simulink model "LKATestBenchExample_sthBrokeGoddamned"  (R2020b)
settings: Solver=FixedStepAuto  StartTime=0.0  StopTime=simStopTime  RelTol=1e-3
PostLoadFcn:
  | helperLKASetUp
values from neighbouring files (symbols this model uses):
  lr = 1.2    [Model_Init.m]    (also in Model_Init_Varying.m; helperLKASetUp.m = 1.6; helperLKASetUpVarying.m = 1.6; modelInit.m)
  m = 1575    [Model_Init.m]    (also in Model_Init_Varying.m; helperLKASetUp.m; helperLKASetUpVarying.m; modelInit.m)
  v = 20    [LVI_PDNN_for_QP_init.m]    (also in Model_Init_Varying.m = 15; automatedBayes.m = i; runSimOnce.m = 36)
  v0_ego = Vx    [Model_Init.m]    (also in Model_Init_Varying.m = 15)
  yaw0_ego = 0    [BayesOpt.m]    (also in helperLKASetUpVarying.m = -90)
undefined symbols (not defined in the file or in its folder): Curvature, CurvatureDerivative, driverPath, driving, HeadingAngle, LateralOffset, Left, Right, Strength
libraries: simulink x2, drivingscenarioandsensors x2, pid_lib x1, autolibshared x1
CloseFcn:
  | helperLKACleanUp
settings Model: Creator=The MathWorks, Inc.  LastModifiedBy=Stage
settings DataIOCC: ReturnWorkspaceOutputs=off
settings DebuggingCC: ParameterPrecisionLossMsg=none  ArithmeticOperatorsInVariantConditions=warning
settings HardwareCC: ProdLongLongMode=on
settings SFSimCC: SimUseLocalCustomCode=off
settings RTWCC: RTWUseLocalCustomCode=off

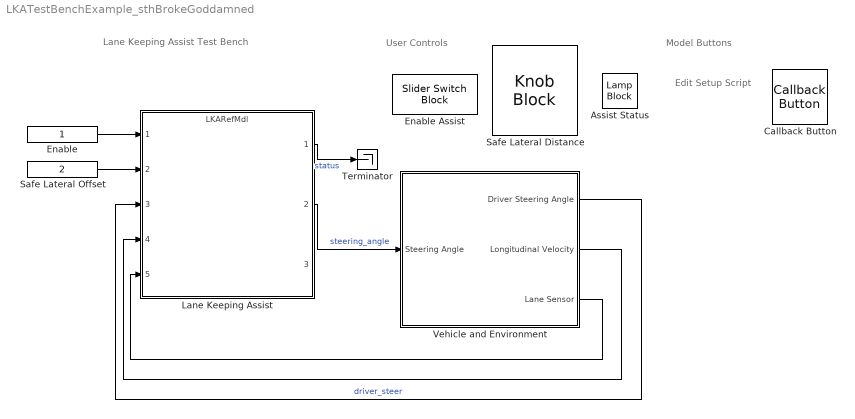
== system LKATestBenchExample_sthBrokeGoddamned ==
  note: User Controls
  note: Edit Setup Script
  note: Lane Keeping Assist Test Bench
  note: Model Buttons
  Assist Status : LampBlock  LabelPosition=Hide
  Callback Button : CallbackButton  ButtonText=?
      settings: ClickFcn=|
      | exampleID = 'LaneKeepingAssistWithLaneDetectionExample';
      | exampleName = 'lane-keeping-assist-with-lane-detection.html';
      | if license('test','automated_driving_toolbox') && ~isempty(ver('driving'))
      |     helpview('driving',exampleID);
      | elseif license('test','MPC_Toolbox') && ~isempty(ver('mpc'))
      |     helpview('mpc',exampleID);
      | else
      |     web(fullfile('https://www.mathworks.com/help','driving','examples',exampleName));
      | end
      | clear exampleName exampleID;
  Enable : Constant  OutDataTypeStr=Inherit: Inherit via back propagation
  Enable Assist : SliderSwitchBlock  LabelPosition=Hide
      settings: Values={{'Off', 'On'}, [0 1]}
  Lane Keeping Assist : ModelReference  ModelNameDialog=LKARefMdl.slx  SimulationMode=Normal  CodeInterface=Top model  ModelReferenceVersion=1.373
  Safe Lateral Distance : KnobBlock  LabelPosition=Hide  ScaleMax=2  TickInterval=0.5
  Safe Lateral Offset : Constant  Value=2  OutDataTypeStr=Inherit: Inherit via back propagation
  Terminator : Terminator
  Vehicle and Environment : Subsystem
  wires:
  Lane Keeping Assist/1 -> Terminator/1  "status"
  Lane Keeping Assist/2 -> Vehicle and Environment/1(Steering Angle)  "steering_angle"
  Enable/1 -> Lane Keeping Assist/1
  Vehicle and Environment/3(Lane Sensor) -> Lane Keeping Assist/5
  Safe Lateral Offset/1 -> Lane Keeping Assist/2
  Vehicle and Environment/1(Driver Steering Angle) -> Lane Keeping Assist/3  "driver_steer"
  Vehicle and Environment/2(Longitudinal Velocity) -> Lane Keeping Assist/4

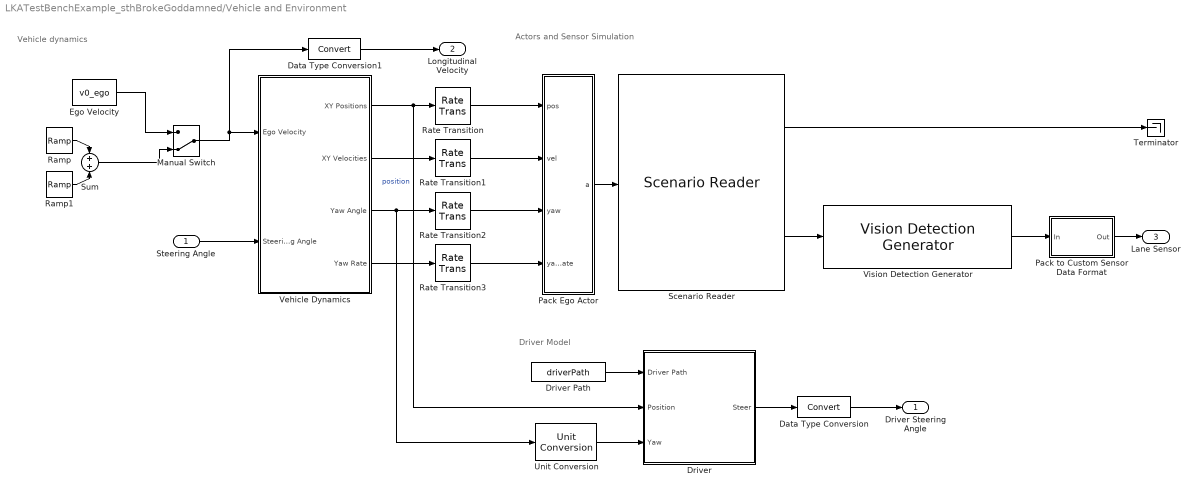
== system LKATestBenchExample_sthBrokeGoddamned/Vehicle and Environment ==
  note: Vehicle dynamics
  note: Actors and Sensor Simulation
  note: Driver Model
  Steering Angle : Inport  Unit=rad
  Data Type Conversion : DataTypeConversion
  Data Type Conversion1 : DataTypeConversion
  Driver : Subsystem
  Driver Path : Constant  Value=driverPath
  Ego Velocity : Constant  Value=v0_ego
  Manual Switch : ManualSwitch  CurrentSetting=0
  Pack Ego Actor : MATLAB Function  TreatAsAtomicUnit=on
  Pack to Custom Sensor Data Format : Subsystem
  Ramp : simulink/Sources/Ramp  slope=-5  start=v/5  InitialOutput=0
  Ramp1 : simulink/Sources/Ramp  slope=5  start=0  InitialOutput=0
  Rate Transition{,1..3} (4 alike) : RateTransition  OutPortSampleTime=Ts
  Scenario Reader : drivingscenarioandsensors/Scenario Reader  ScenarioSource=From workspace  ScenarioFileName=MyDynamicScenario.mat  ScenarioVariableName=scenario1  OutputCoordinateSystem=Vehicle coordinates  EgoVehicleSource=Input port  EgoVehicleActorID=1  OrientVehiclesOnRoad=off  OutputEgoVehiclePose=off  SampleTime=0.1  LaneBoundaryOutput=Ego vehicle lane boundaries  LaneBoundaryDistance=0:0.5:60  LaneBoundaryLocation=Inner edge of lane markings  BusNameSource=Auto  BusName=BusActors  BusName2Source=Auto  BusName2=BusLaneBoundaries  BusName3Source=Auto  BusName3=BusEgoActor  ShowCoordinateLabels=on  SimulateUsing=Interpreted execution
  Sum : Sum  Inputs=+|+
  Terminator : Terminator
  Unit Conversion : UnitConversion
  Vehicle Dynamics : Subsystem  VariantControl=VariantVDBS
  Vision Detection Generator : drivingscenarioandsensors/Vision Detection Generator  SensorIndex=1  DetectorOutput=Lanes only  UpdateInterval=0.1  LaneUpdateInterval=0.1  SensorLocation=[ 1.9, 0 ]  Height=1.1  Yaw=0  Pitch=1  Roll=0  BusNameSource=Auto  BusName=BusObjectDetections  BusName2Source=Property  BusName2=BusVision  MaxNumDetectionsSource=Property  MaxNumDetections=50  MaxNumLanesSource=Property  MaxNumLanes=2  DetectionCoordinates=Ego Cartesian  SimulateUsing=Interpreted execution  MaxRange=150  BoundingBoxAccuracy=5  ProcessNoiseIntensity=5  MaxSpeed=50  MaxAllowedOcclusion=0.5  MinObjectImageSize=[ 15, 15 ]  DetectionProbability=0.9  FalsePositivesPerImage=0.1  MinLaneImageSize=[ 20, 3 ]  LaneBoundaryAccuracy=3  HasNoise=on  InitialSeedSource=Repeatable  InitialSeed=0  UsedSeed=driving.internal.SimulinkUtilities.seedManager(gcb)  ActorProfilesSource=Parameters  ActorProfilesParameters=driving.internal.ActorProfilesParameters  ActorProfilesExpression=struct( 'ClassID', 0, 'Length', 4.7, 'Width', 1.8, 'Height', 1.4, 'OriginOffset', [ -1.35, 0, 0 ] )  Intrinsics=driving.internal.cameraIntrinsics('FocalLength',[ 100, 100 ])
  Driver Steering Angle : Outport  VectorParamsAs1DForOutWhenUnconnected=off
  Longitudinal Velocity : Outport  Port=2  OutDataTypeStr=single  Unit=m/s  VectorParamsAs1DForOutWhenUnconnected=off
  Lane Sensor : Outport  Port=3  VectorParamsAs1DForOutWhenUnconnected=off
  wires:
  Scenario Reader/1 -> Terminator/1
  Pack Ego Actor/1(a) -> Scenario Reader/1
  Vehicle Dynamics/2(XY Velocities) -> Rate Transition1/1
  Vehicle Dynamics/3(Yaw Angle) -> Unit Conversion/1, Rate Transition2/1
  Rate Transition/1 -> Pack Ego Actor/1(pos)
  Vehicle Dynamics/4(Yaw Rate) -> Rate Transition3/1
  Rate Transition2/1 -> Pack Ego Actor/3(yaw)
  Rate Transition1/1 -> Pack Ego Actor/2(vel)
  Rate Transition3/1 -> Pack Ego Actor/4(yawRate)
  Scenario Reader/2 -> Vision Detection Generator/1
  Vehicle Dynamics/1(XY Positions) -> Driver/2(Position), Rate Transition/1  "position"
  Driver/1(Steer) -> Data Type Conversion/1
  Steering Angle/1 -> Vehicle Dynamics/2(Steering Angle)
  Unit Conversion/1 -> Driver/3(Yaw)
  Vision Detection Generator/1 -> Pack to Custom Sensor Data Format/1(In)
  Data Type Conversion/1 -> Driver Steering Angle/1
  Pack to Custom Sensor Data Format/1(Out) -> Lane Sensor/1
  Data Type Conversion1/1 -> Longitudinal Velocity/1
  Driver Path/1 -> Driver/1(Driver Path)
  Ramp1/1 -> Sum/2
  Ramp/1 -> Sum/1
  Ego Velocity/1 -> Manual Switch/1
  Manual Switch/1 -> Data Type Conversion1/1, Vehicle Dynamics/1(Ego Velocity)
  Sum/1 -> Manual Switch/2

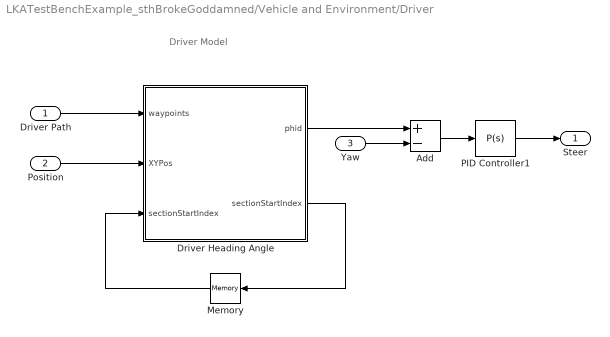
== system LKATestBenchExample_sthBrokeGoddamned/Vehicle and Environment/Driver ==
  note: Driver Model
  Driver Path : Inport  Unit=m
  Position : Inport  Port=2  Unit=m
  Yaw : Inport  Port=3  Unit=rad
  Add : Sum  Inputs=+-
  Driver Heading Angle : MATLAB Function  TreatAsAtomicUnit=on
  Memory : Memory
  PID Controller1 : pid_lib/PID Controller  Controller=P  Form=Parallel  TimeDomain=Continuous-time  UseExternalTs=off  SampleTime=-1  IntegratorMethod=Forward Euler  FilterMethod=Forward Euler  ControllerParametersSource=internal  P=1  I=0.002  D=0.00001  UseFilter=on  N=100  TunerSelectOption=Transfer Function Based (PID Tuner App)  InitialConditionSource=internal  InitialConditionForIntegrator=0  InitialConditionForFilter=0  DifferentiatorICPrevScaledInput=0  ExternalReset=none  TrackingMode=off  Kt=1  LimitOutput=off  SatLimitsSource=internal  UpperSaturationLimit=inf  LowerSaturationLimit=-inf  LinearizeAsGain=on  AntiWindupMode=none  Kb=1  POutMin=[]  POutMax=[]  IOutMin=[]  IOutMax=[]  DOutMin=[]  DOutMax=[]  NOutMin=[]  NOutMax=[]  SumOutMin=[]  SumOutMax=[]  SaturationOutMin=[]  SaturationOutMax=[]  PParamMin=[]  PParamMax=[]  IParamMin=[]  IParamMax=[]  DParamMin=[]  DParamMax=[]  NParamMin=[]  NParamMax=[]  KbParamMin=[]  KbParamMax=[]  KtParamMin=[]  KtParamMax=[]  KbOutMin=[]  KbOutMax=[]  KtOutMin=[]  KtOutMax=[]  IntegratorOutMin=[]  IntegratorOutMax=[]  FilterOutMin=[]  FilterOutMax=[]  SumI1OutMin=[]  SumI1OutMax=[]  SumI2OutMin=[]  SumI2OutMax=[]  SumI3OutMin=[]  SumI3OutMax=[]  SumI4OutMin=[]  SumI4OutMax=[]  SumDOutMin=[]  SumDOutMax=[]  DifferentiatorOutMin=[]  DifferentiatorOutMax=[]  FilterDiffOutCoefMin=[]  FilterDiffOutCoefMax=[]  ReciprocalOutMin=[]  ReciprocalOutMax=[]  SumDenOutMin=[]  SumDenOutMax=[]  SumNumOutMin=[]  SumNumOutMax=[]  DivideOutMin=[]  DivideOutMax=[]  UdiffTsProdOutMin=[]  UdiffTsProdOutMax=[]  NTsProdOutMin=[]  NTsProdOutMax=[]  UintegralTsProdOutMin=[]  UintegralTsProdOutMax=[]  UngainTsProdOutMin=[]  UngainTsProdOutMax=[]  IntegratorContinuousStateAttributes=''  IntegratorStateMustResolveToSignalObject=off  IntegratorRTWStateStorageClass=Auto  FilterContinuousStateAttributes=''  FilterStateMustResolveToSignalObject=off  FilterRTWStateStorageClass=Auto  ParallelPVariant=InternalParameters  IdealPVariant=Disabled  IVariant=Disabled  DVariant=Disabled  IntegratorVariant=Disabled  SatVariant=Disabled  AWVariant=Disabled  PCopyVariant=Disabled  TRVariant=Disabled  FdbkBlocksVariant=Forward  IdealPFdbkVariant=Disabled  SatFdbkVariant=Disabled  DerivativeFilterVariant=Disabled  NVariant=Disabled  NCopyVariant=Disabled_SignalSpec  FilterICVariant=Disabled  IntegratorICVariant=Disabled  ExternalResetVariant=Disabled  TRSumVariant=Passthrough  SumFdbkVariant=Disabled  SumVariant=Passthrough_P  TsampFilterVariant=InternalTs  TsampNgainVariant=Passthrough  TsampIntegralVariant=Disabled_SignalSpec  ExternalSaturationOutDataTypeStr=Inherit: Same as second input
  Steer : Outport  Unit=rad  VectorParamsAs1DForOutWhenUnconnected=off
  wires:
  Yaw/1 -> Add/2
  Position/1 -> Driver Heading Angle/2(XYPos)
  Driver Path/1 -> Driver Heading Angle/1(waypoints)
  Driver Heading Angle/1(phid) -> Add/1
  PID Controller1/1 -> Steer/1
  Driver Heading Angle/2(sectionStartIndex) -> Memory/1
  Memory/1 -> Driver Heading Angle/3("sectionStartIndex ")
  Add/1 -> PID Controller1/1

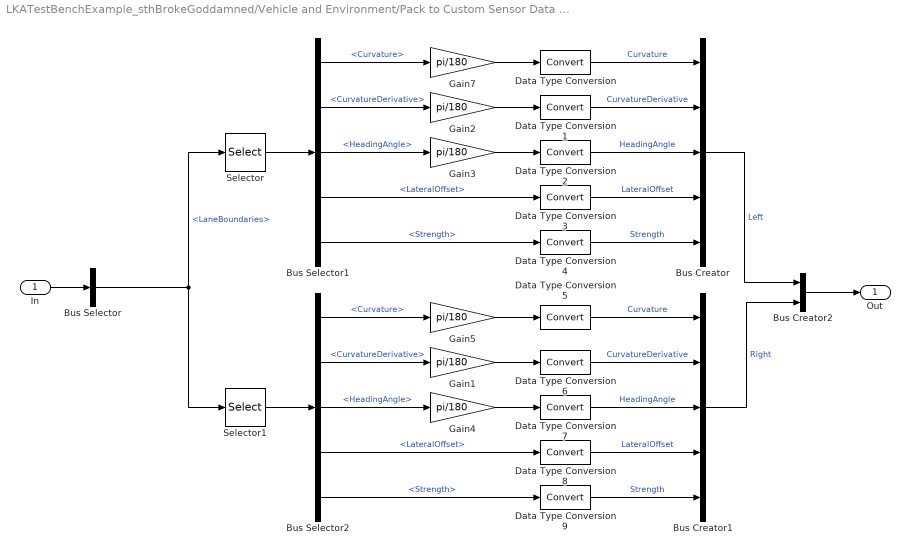
== system LKATestBenchExample_sthBrokeGoddamned/Vehicle and Environment/Pack to Custom Sensor Data Format ==
  In : Inport
  Bus Creator : BusCreator  Inputs=Curvature,CurvatureDerivative,HeadingAngle,LateralOffset,Strength  OutDataTypeStr=Bus: LaneSensorBoundaries
  Bus Creator1 : BusCreator  Inputs=Curvature,CurvatureDerivative,HeadingAngle,LateralOffset,Strength  OutDataTypeStr=Bus: LaneSensorBoundaries
  Bus Creator2 : BusCreator  Inputs=Left,Right  OutDataTypeStr=Bus: LaneSensor
  Bus Selector : BusSelector  OutputSignals=LaneBoundaries
  Bus Selector1 : BusSelector  OutputSignals=Curvature,CurvatureDerivative,HeadingAngle,LateralOffset,Strength
  Bus Selector2 : BusSelector  OutputSignals=Curvature,CurvatureDerivative,HeadingAngle,LateralOffset,Strength
  Data Type Conversion{,1..9} (10 alike) : DataTypeConversion
  Gain{1..5,7} (6 alike) : Gain  Gain=pi/180
  Selector : Selector  InputPortWidth=2  IndexOptions=Index vector (dialog)  Indices=1  OutputSizes=1
  Selector1 : Selector  InputPortWidth=2  IndexOptions=Index vector (dialog)  Indices=2  OutputSizes=1
  Out : Outport  VectorParamsAs1DForOutWhenUnconnected=off
  wires:
  In/1 -> Bus Selector/1
  Bus Selector/1 -> Selector/1, Selector1/1  "<LaneBoundaries>"
  Selector/1 -> Bus Selector1/1
  Bus Selector1/2 -> Gain2/1  "<CurvatureDerivative>"
  Bus Selector1/1 -> Gain7/1  "<Curvature>"
  Bus Selector1/3 -> Gain3/1  "<HeadingAngle>"
  Gain7/1 -> Data Type Conversion/1
  Gain2/1 -> Data Type Conversion1/1
  Gain3/1 -> Data Type Conversion2/1
  Bus Selector1/4 -> Data Type Conversion3/1  "<LateralOffset>"
  Bus Selector1/5 -> Data Type Conversion4/1  "<Strength>"
  Data Type Conversion/1 -> Bus Creator/1  "Curvature"
  Data Type Conversion1/1 -> Bus Creator/2  "CurvatureDerivative"
  Data Type Conversion2/1 -> Bus Creator/3  "HeadingAngle"
  Data Type Conversion3/1 -> Bus Creator/4  "LateralOffset"
  Data Type Conversion4/1 -> Bus Creator/5  "Strength"
  Data Type Conversion9/1 -> Bus Creator1/5  "Strength"
  Data Type Conversion6/1 -> Bus Creator1/2  "CurvatureDerivative"
  Data Type Conversion7/1 -> Bus Creator1/3  "HeadingAngle"
  Data Type Conversion8/1 -> Bus Creator1/4  "LateralOffset"
  Data Type Conversion5/1 -> Bus Creator1/1  "Curvature"
  Bus Selector2/1 -> Gain5/1  "<Curvature>"
  Selector1/1 -> Bus Selector2/1
  Bus Selector2/4 -> Data Type Conversion8/1  "<LateralOffset>"
  Bus Selector2/5 -> Data Type Conversion9/1  "<Strength>"
  Bus Selector2/2 -> Gain1/1  "<CurvatureDerivative>"
  Gain4/1 -> Data Type Conversion7/1
  Gain5/1 -> Data Type Conversion5/1
  Gain1/1 -> Data Type Conversion6/1
  Bus Selector2/3 -> Gain4/1  "<HeadingAngle>"
  Bus Creator2/1 -> Out/1
  Bus Creator/1 -> Bus Creator2/1  "Left"
  Bus Creator1/1 -> Bus Creator2/2  "Right"

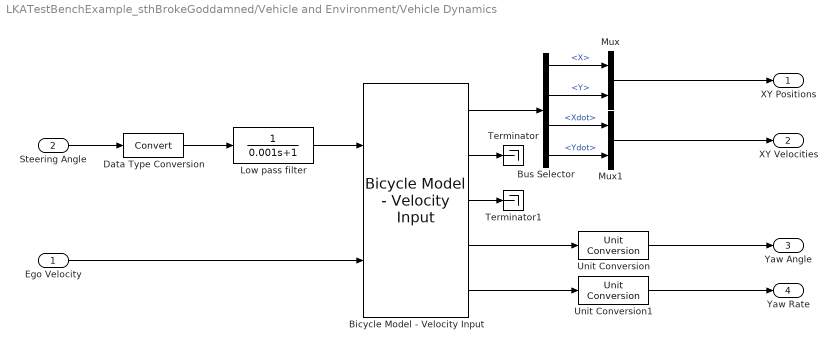
== system LKATestBenchExample_sthBrokeGoddamned/Vehicle and Environment/Vehicle Dynamics ==
  Ego Velocity : Inport
  Steering Angle : Inport  Port=2
  Bicycle Model - Velocity Input : autolibshared/Bicycle Model - Velocity Input  trackMode=Single (bicycle)  inputMode=External longitudinal forces  frontSteerMode=on  rearSteerMode=off  windMode=off  muMode=off  extFMode=off  extMMode=off  aMode=3  NF=2  NR=2  m=m  a=lf  b=lr  h=0.35  X_o=x0_ego  xdot_o=0  CalphaMode=off  sigmaMode=on  w=[1.4,1.4]  Cy_f=Cf  Cy_r=Cr  sigma_f=.1  sigma_r=.1  alpha_f_brk=[-.1 .1]  Cy_f_data=[-9e3 9e3]  alpha_r_brk=[-.1 .1]  Cy_r_data=[-9e3 9e3]  Y_o=y0_ego  ydot_o=0  Izz=Iz  psi_o=yaw0_ego*pi/180  r_o=0  Af=0  Cd=0  Cl=0  Cpm=0  beta_w=[0:0.0001:0.003]  Cs=[0:0.0003:0.009]  Cym=[0:0.0001:0.003]  Pabs=101325  Tair=273  g=9.81  mu=1  xdot_tol=.01  Fznom=5000  Fxtire_sat=1e6  Fytire_sat=1e6  longOff=0  latOff=0  vertOff=0
      settings: SourceProductBaseCode=PW,MT,UV,VE,VP
  Bus Selector : BusSelector  OutputSignals=InertFrm.FrntAxl.Disp.X,InertFrm.FrntAxl.Disp.Y,InertFrm.FrntAxl.Vel.Xdot,InertFrm.FrntAxl.Vel.Ydot
  Data Type Conversion : DataTypeConversion
  Low pass filter : TransferFcn  Denominator=[0.001 1]
  Mux : Mux  Inputs=2
  Mux1 : Mux  Inputs=2
  Terminator : Terminator
  Terminator1 : Terminator
  Unit Conversion : UnitConversion  OutputType=Inherit: Inherit via back propagation
  Unit Conversion1 : UnitConversion  OutputType=Inherit: Inherit via back propagation
  XY Positions : Outport  Unit=m  VectorParamsAs1DForOutWhenUnconnected=off
  XY Velocities : Outport  Port=2  Unit=m/s  VectorParamsAs1DForOutWhenUnconnected=off
  Yaw Angle : Outport  Port=3  Unit=deg  VectorParamsAs1DForOutWhenUnconnected=off
  Yaw Rate : Outport  Port=4  Unit=degree/s  VectorParamsAs1DForOutWhenUnconnected=off
  wires:
  Mux/1 -> XY Positions/1
  Mux1/1 -> XY Velocities/1
  Unit Conversion1/1 -> Yaw Rate/1
  Unit Conversion/1 -> Yaw Angle/1
  Ego Velocity/1 -> Bicycle Model - Velocity Input/2
  Bicycle Model - Velocity Input/1 -> Bus Selector/1
  Bicycle Model - Velocity Input/2 -> Terminator/1
  Bicycle Model - Velocity Input/3 -> Terminator1/1
  Bicycle Model - Velocity Input/4 -> Unit Conversion/1
  Bicycle Model - Velocity Input/5 -> Unit Conversion1/1
  Bus Selector/1 -> Mux/1  "<X>"
  Bus Selector/2 -> Mux/2  "<Y>"
  Bus Selector/3 -> Mux1/1  "<Xdot>"
  Bus Selector/4 -> Mux1/2  "<Ydot>"
  Data Type Conversion/1 -> Low pass filter/1
  Steering Angle/1 -> Data Type Conversion/1
  Low pass filter/1 -> Bicycle Model - Velocity Input/1

== matlab function LKATestBenchExample_sthBrokeGoddamned/Vehicle and Environment/Pack Ego Actor ==
  data: pos input; a output Bus: BusActors1Actors size=1; vel input; yaw input; yawRate input
function a = packEgo(pos,vel,yaw,yawRate)
% Pack ego information into a single ego actor bus
%
% Imoprtant note:
% Output is a bus of type BusActorsActors. This is the same bus used by the
% Scenario Reader to output an individual actor. If you change the
% output bus name of Scenario Reader change the output bus name here
% as well by clicking on 'Edit Data' in the menu above.

a = struct(...
    'ActorID',1,...
    'Position', [pos(1) pos(2) 0], ...
    'Velocity', [vel(1) vel(2) 0], ...
    'Roll', 0, ...
    'Pitch', 0, ...
    'Yaw', yaw, ...
    'AngularVelocity', [0 0 yawRate]);

== matlab function LKATestBenchExample_sthBrokeGoddamned/Vehicle and Environment/Driver/Driver Heading Angle ==
  data: waypoints input; XYPos input; phid output; sectionStartIndex input; sectionStartIndex output
function [phid,sectionStartIndex] = driverHeadingAngle(waypoints, XYPos, sectionStartIndex)
% DRIVERHEADINGANGLE
% XYPos     = Current position of vehicle
% waypoints = Desired path
% phid      = Desired heading angle

if sectionStartIndex < 1
    sectionStartIndex = 1;
end

numWaypoints = size(waypoints,1);

% Distance between section start and end points
DeltaXY = [waypoints(sectionStartIndex+1,1)-waypoints(sectionStartIndex,1),...
           waypoints(sectionStartIndex+1,2)-waypoints(sectionStartIndex,2)];

% Distance between current position and section starting point
RXY = [XYPos(1)-waypoints(sectionStartIndex,1),...
       XYPos(2)-waypoints(sectionStartIndex,2)];

% Normalized distance between current position and section starting point
u = (RXY.*DeltaXY)/(DeltaXY.*DeltaXY);

% Find section ending point
indexIncrement = ceil(u-1);

if indexIncrement<0
    % In current section
    indexIncrement = 0;
end
if u >=1
    % Increment to appropriate section 
    % with the assumption that the distance between waypoints is 
    % approximately equal for near sections
    sectionStartIndex = sectionStartIndex+indexIncrement;
    % Adjust u to account for new section starting point
    u = u - indexIncrement;
end


if sectionStartIndex < (numWaypoints-1)
    % Operating within valid sections
    currentSectionEndIndex = sectionStartIndex+1;
    nextSectionEndIndex    = currentSectionEndIndex+1;

    % Target position at end point of current and next sections
    XYTarget1 = [waypoints(currentSectionEndIndex,1),...
                 waypoints(currentSectionEndIndex,2)];
    XYTarget2 = [waypoints(nextSectionEndIndex,1),...
                 waypoints(nextSectionEndIndex,2)];
    % Section weights         
    Weight1 = (1-u);
    Weight2 = u;

    % Target position
    XYTarget = Weight1*XYTarget1+Weight2*XYTarget2;
    
    % Desired heading
    phid = atan2((XYTarget(2)-XYPos(2)),...
                 (XYTarget(1)-XYPos(1)));
else
    % Maintain last heading between points
    sectionStartIndex = numWaypoints-1;
    phid = atan2((waypoints(end,2)-waypoints(end-1,2)),...
                 (waypoints(end,1)-waypoints(end-1,1)));
end
